simulink model "sim1"  (R2024a)
settings: Solver=VariableStepAuto  StartTime=0.0  StopTime=10.0  FixedStep=1e-3  RelTol=1e-3
InitFcn:
  | A=[7 -4;
  |     5 6];
  | B=[5;
  |     2];
  | Bf=[3;
  |     9];
  | Q=[3 0;
  |     0 4];
  | K=[4.459819386505104e+04,-5.046739138317868e+05];
settings Model: Creator=alexe  LastModifiedBy=alexe

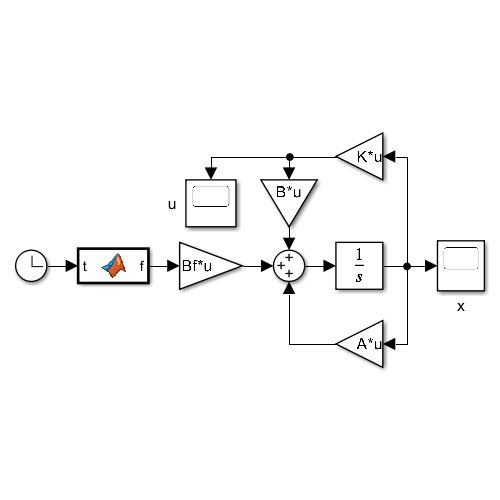
[thumbnail: Simulink's stored preview of the top-level diagram]
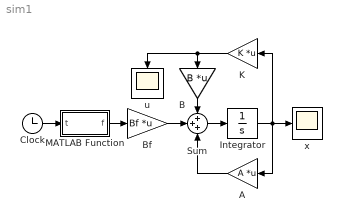
== system sim1 ==
  A : Gain  Gain=A  Multiplication=Matrix(K*u)
  B : Gain  Gain=B  Multiplication=Matrix(K*u)
  Bf : Gain  Gain=Bf  Multiplication=Matrix(K*u)
  Clock : Clock
  Integrator : Integrator  InitialCondition=[1;0];
  K : Gain  Gain=K  Multiplication=Matrix(K*u)
  MATLAB Function : MATLAB Function  TreatAsAtomicUnit=on
  Sum : Sum  Inputs=+++
  u : Scope
  x : Scope
  wires:
  Integrator/1 -> x/1, K/1, A/1
  A/1 -> Sum/3
  Sum/1 -> Integrator/1
  Bf/1 -> Sum/2
  Clock/1 -> MATLAB Function/1(t)
  MATLAB Function/1(f) -> Bf/1
  K/1 -> u/1, B/1
  B/1 -> Sum/1

== matlab function sim1/MATLAB Function ==
  data: t input; f output
function f = fcn(t)

f = 10*sin(6*t)+5*cos(2*t)+4*cos(3*t)+3*cos(8*t);
